simulink model "SMIB_with_DFIG_IO"  (R2016a)
settings: Solver=ode4  StartTime=0.0  StopTime=10  FixedStep=0.01  RelTol=1e-3
values from neighbouring files (symbols this model uses):
  d_base = 5.0009990    (= 5.000999)    [find_dfig_state_initial_conditions.m]
  d_Beta = 0    [find_dfig_state_initial_conditions.m]
  d_bl = 40.0595545    [find_dfig_state_initial_conditions.m]
  d_Cdc = 2    [find_dfig_state_initial_conditions.m]
  d_Cf = d_FLTR(6)    [find_dfig_state_initial_conditions.m]
  d_ctg = 0.01    [Initialising_SMIB_DFIG.m]    (also in Initialising_two_area_DFIG.m; find_dfig_state_initial_conditions.m = data_DF(10))
  d_esd = -d_Kmrr.*d_ws.*(d_Lrr.*d_irq + d_Lm.*d_isq)    [find_dfig_state_initial_conditions.m]
  d_esq = d_Kmrr.*d_ws.*(d_Lrr.*d_ird + d_Lm.*d_isd)    [find_dfig_state_initial_conditions.m]
  d_GSC_IL1_iv = real(d_vi_dash)    [find_dfig_state_initial_conditions.m]
  d_GSC_IL1_kp = 0.3    [Initialising_SMIB_DFIG.m]    (also in Initialising_two_area_DFIG.m)
  d_GSC_IL2_iv = imag(d_vi_dash)    [find_dfig_state_initial_conditions.m]
  d_GSC_IL2_kp = 0.3    [Initialising_SMIB_DFIG.m]    (also in Initialising_two_area_DFIG.m)
  d_GSC_OL1_iv = real(d_ii_dash)    [find_dfig_state_initial_conditions.m]
  d_GSC_OL1_kp = -22    [Initialising_SMIB_DFIG.m]    (also in Initialising_two_area_DFIG.m)
  d_GSC_OL2_iv = imag(d_ii_dash)    [find_dfig_state_initial_conditions.m]
  d_GSC_OL2_kp = 0    [Initialising_SMIB_DFIG.m]    (also in Initialising_two_area_DFIG.m)
  d_Hg = 0.4    [Initialising_SMIB_DFIG.m]    (also in Initialising_two_area_DFIG.m; find_dfig_state_initial_conditions.m = data_DF(12))
  d_Ht = 4    [Initialising_SMIB_DFIG.m]    (also in Initialising_two_area_DFIG.m; find_dfig_state_initial_conditions.m = data_DF(11))
  d_igd = xdfig(:,10)    [find_dfig_state_initial_conditions.m]
  d_igq = xdfig(:,9)    [find_dfig_state_initial_conditions.m]
  d_iid = xdfig(:,8)    [find_dfig_state_initial_conditions.m]
  d_iiq = xdfig(:,7)    [find_dfig_state_initial_conditions.m]
  d_isd = xdfig(:,2)    [find_dfig_state_initial_conditions.m]
  d_isq = xdfig(:,1)    [find_dfig_state_initial_conditions.m]
  d_Kmrr = d_Lm/d_Lrr    [find_dfig_state_initial_conditions.m]
  d_Kopt = 1    [Initialising_SMIB_DFIG.m]    (also in Initialising_two_area_DFIG.m; find_dfig_state_initial_conditions.m = data_DF(8))
  d_ktg = 0.3    [Initialising_SMIB_DFIG.m]    (also in Initialising_two_area_DFIG.m)
  d_Lg = d_FLTR(5)    [find_dfig_state_initial_conditions.m]
  d_Li = d_FLTR(4)    [find_dfig_state_initial_conditions.m]
  d_Lm = 4    [Initialising_SMIB_DFIG.m]    (also in Initialising_two_area_DFIG.m; find_dfig_state_initial_conditions.m = data_DF(3))
  d_Ls_d = d_Lss - (d_Lm^2/d_Lrr)    [find_dfig_state_initial_conditions.m]
  d_MSC_IL1_iv = 0.0389    [Initialising_SMIB_DFIG.m]    (also in Initialising_two_area_DFIG.m; find_dfig_state_initial_conditions.m = real(d_vr_dash))
  d_MSC_IL1_kp = -0.23    [Initialising_SMIB_DFIG.m]    (also in Initialising_two_area_DFIG.m)
  d_MSC_IL2_iv = imag(d_vr_dash)    [find_dfig_state_initial_conditions.m]
  d_MSC_IL2_kp = -0.23    [Initialising_SMIB_DFIG.m]    (also in Initialising_two_area_DFIG.m)
  d_MSC_OL1_iv = real(d_ir_dash)    [find_dfig_state_initial_conditions.m]
  d_MSC_OL1_kp = 0    [Initialising_SMIB_DFIG.m]    (also in Initialising_two_area_DFIG.m)
  d_MSC_OL2_iv = imag(d_ir_dash)    [find_dfig_state_initial_conditions.m]
  d_MSC_OL2_kp = 0    [Initialising_SMIB_DFIG.m]    (also in Initialising_two_area_DFIG.m)
  d_Qs = Qdfig    [find_dfig_state_initial_conditions.m]
  d_R1 = d_Rs + d_R2    [find_dfig_state_initial_conditions.m]
  d_R2 = d_Kmrr^2*d_Rr    [find_dfig_state_initial_conditions.m]
  d_Rc = d_FLTR(3)    [find_dfig_state_initial_conditions.m]
  d_Rg = 0.0    (= 0)    [find_dfig_state_initial_conditions.m]
  d_Ri = 0.0    (= 0)    [find_dfig_state_initial_conditions.m]
  d_Tr = d_Lrr/d_Rr    [find_dfig_state_initial_conditions.m]
  d_Ts = 0.9386    [find_dfig_state_initial_conditions.m]
  d_vcd = xdfig(:,14)    [find_dfig_state_initial_conditions.m]
  d_vcq = 0.9837    [Initialising_SMIB_DFIG.m]    (also in Initialising_two_area_DFIG.m)
  d_VDC = 1.5    [find_dfig_state_initial_conditions.m]
  d_vw = 14.5316    [Initialising_SMIB_DFIG.m]    (also in Initialising_two_area_DFIG.m; find_dfig_state_initial_conditions.m)
  d_wb = 2*pi*50    (= 314.159265359)    [Initialising_SMIB_DFIG.m]    (also in Initialising_two_area_DFIG.m; find_dfig_state_initial_conditions.m)
  d_welb = 2*pi*50    (= 314.159265359)    [find_dfig_state_initial_conditions.m]
  d_wg = 0.9688    [find_dfig_state_initial_conditions.m]
  d_ws = 1    [Initialising_SMIB_DFIG.m]    (also in Initialising_two_area_DFIG.m; find_dfig_state_initial_conditions.m)
  d_wt = 0.9688    [find_dfig_state_initial_conditions.m]
  d_wtrated = 3.0337    [find_dfig_state_initial_conditions.m]
  d_Xm = d_Lm    [find_dfig_state_initial_conditions.m]
  dfig_mult = zeros(size(bus_sln,1)-1,size(Dmachs,1))    [Initialising_SMIB_DFIG.m]    (also in Initialising_two_area_DFIG.m)
  ExpandSmachs = [1]    [Initialising_SMIB_DFIG.m]    (also in Initialising_two_area_DFIG.m)
  MMST_mult = zeros(size(bus_sln,1)-1,size(Smachs,1))    [Initialising_SMIB_DFIG.m]    (also in Initialising_two_area_DFIG.m)
  rho = 1.225    [find_dfig_state_initial_conditions.m]
  s_delta = s_delta*(180/pi)    [Initialising_SMIB_DFIG.m]    (also in Initialising_two_area_DFIG.m; generic_Sync_Init.m = angle(s_Eq))
  s_Edd = -(s_xq-s_xqd).* s_iq    [generic_Sync_Init.m]
  s_Efd = abs(s_Eq) - (s_xd-s_xq).*s_id    [generic_Sync_Init.m]
  s_Eqd = s_Efd + (s_xd-s_xdd).*s_id    [generic_Sync_Init.m]
  s_f = 60    [generic_Sync_Init.m]
  s_Ka = 200    [two_area_synch.m]
  s_Psi2q = -s_Edd+(s_xqd-s_xls).*s_iq    [generic_Sync_Init.m]
  s_Psild = s_Eqd+(s_xdd-s_xls).*s_id    [generic_Sync_Init.m]
  s_Rgov = 0.05    [two_area_synch.m]
  s_Ta = 0.02    [two_area_synch.m]
  s_Tg = 0.2    [two_area_synch.m]
  s_Tm = s_Te    [generic_Sync_Init.m]
  s_Vref = s_volt+1./s_Ka.*s_Efd    [generic_Sync_Init.m]
  s_ws = 0    [generic_Sync_Init.m]
  SelectSmachs = [1]    [Initialising_SMIB_DFIG.m]    (also in Initialising_two_area_DFIG.m)
  small_d = [ ... (first row only)    [Initialising_SMIB_DFIG.m]    (also in Initialising_two_area_DFIG.m; initSSA.m; two_area_synch.m)
  vinf = bus_sln(3,2)*exp(1i*bus_sln(3,3)*pi/180)    [Initialising_SMIB_DFIG.m]    (also in Initialising_two_area_DFIG.m)
  ZA = Znet(1:end-1,1:end-1)    [Initialising_SMIB_DFIG.m]    (also in Initialising_two_area_DFIG.m)
  ZB = Znet(1:end-1,end)    [Initialising_SMIB_DFIG.m]    (also in Initialising_two_area_DFIG.m)
  ZC = Znet(end,1:end-1)    [Initialising_SMIB_DFIG.m]    (also in Initialising_two_area_DFIG.m)
  ZD = Znet(end,end)    [Initialising_SMIB_DFIG.m]    (also in Initialising_two_area_DFIG.m)
undefined symbols (not defined in the file or in its folder): j, s_D, s_H, s_Rs, s_Tdod, s_Tdodd, s_Tqod, s_Tqodd, s_xd, s_xdd, s_xddd, s_xls, s_xq, s_xqd, s_xqdd
libraries: powerlib_extras x1
settings Model: Creator=EBUKA  LastModifiedBy=EBUKA
settings GRTTargetCC: GeneratePreprocessorConditionals=Use local settings

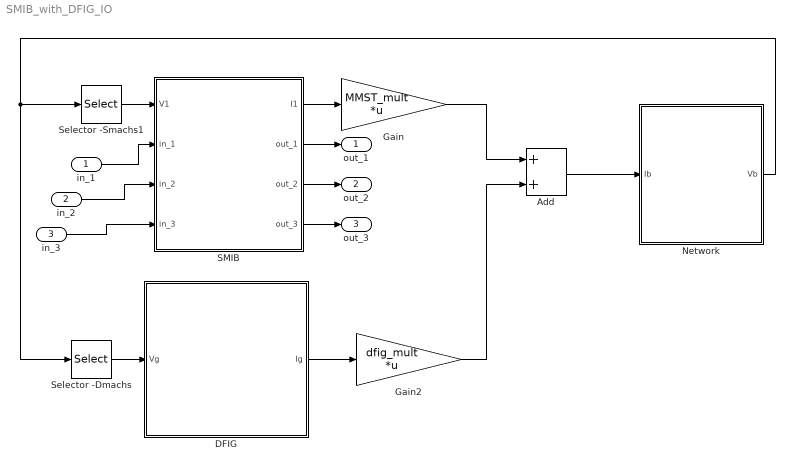
== system SMIB_with_DFIG_IO ==
  in_1 : Inport
  in_2 : Inport  Port=2
  in_3 : Inport  Port=3
  Add : Sum
  DFIG : Subsystem
  Gain : Gain  Gain=MMST_mult  Multiplication=Matrix(K*u)
  Gain2 : Gain  Gain=dfig_mult  Multiplication=Matrix(K*u)
  Network : Subsystem
  SMIB : Subsystem
  Selector -Dmachs : Selector  InputPortWidth=13  IndexOptions=Index vector (dialog)  Indices=Dmachs  OutputSizes=1
  Selector -Smachs1 : Selector  InputPortWidth=13  IndexOptions=Index vector (dialog)  Indices=Smachs  OutputSizes=1
  out_1 : Outport
  out_2 : Outport  Port=2
  out_3 : Outport  Port=3
  wires:
  Selector -Smachs1/1 -> SMIB/1(V1)
  SMIB/1(I1) -> Gain/1
  Add/1 -> Network/1(Ib)
  Gain/1 -> Add/1
  Gain2/1 -> Add/2
  DFIG/1(Ig) -> Gain2/1
  Selector -Dmachs/1 -> DFIG/1(Vg)
  Network/1(Vb) -> Selector -Smachs1/1, Selector -Dmachs/1
  in_1/1 -> SMIB/2(in_1)
  in_2/1 -> SMIB/3(in_2)
  in_3/1 -> SMIB/4(in_3)
  SMIB/2(out_1) -> out_1/1
  SMIB/3(out_2) -> out_2/1
  SMIB/4(out_3) -> out_3/1

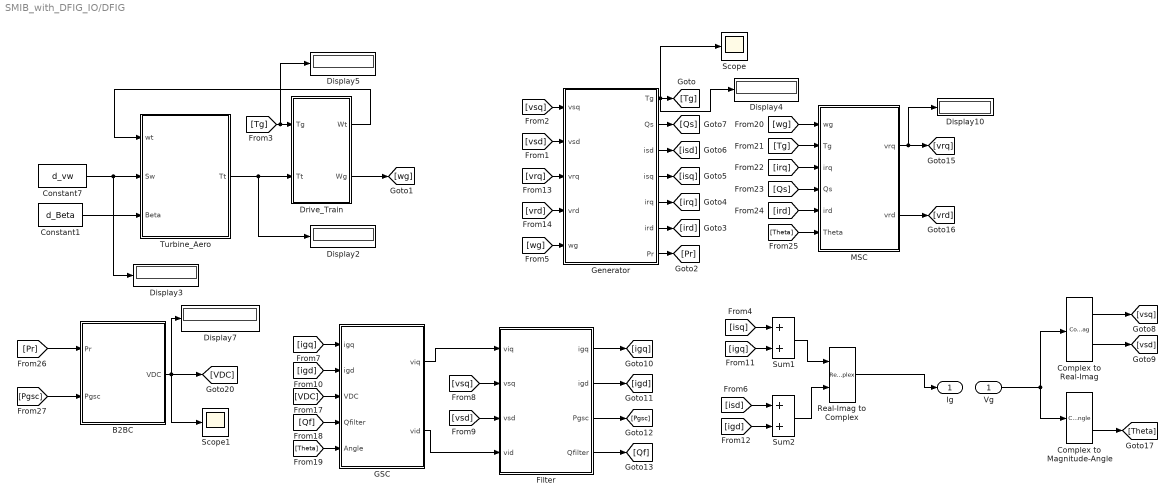
== system SMIB_with_DFIG_IO/DFIG ==
  Vg : Inport
  B2BC : Subsystem
  Complex to Magnitude-Angle : ComplexToMagnitudeAngle
  Complex to Real-Imag : ComplexToRealImag
  Constant1 : Constant  Value=d_Beta
  Constant7 : Constant  Value=d_vw
  Display{2..5,7,10} (6 alike) : Display
  Drive_Train : Subsystem
  Filter : Subsystem
  GSC : Subsystem
  Generator : Subsystem
  MSC : Subsystem
  Real-Imag to Complex : RealImagToComplex
  Scope : Scope
  Scope1 : Scope
  Sum1 : Sum
  Sum2 : Sum
  Turbine_Aero : Subsystem
  Ig : Outport
  wires:
  [vrd] -> Generator/4(vrd)
  [vsd] -> Generator/2(vsd)
  Drive_Train/1(Wt) -> Turbine_Aero/1(wt)
  Generator/6(ird) -> [ird]
  [Tg] -> Display5/1, Drive_Train/1(Tg)
  Constant7/1 -> Display3/1, Turbine_Aero/2(Sw)
  Turbine_Aero/1(Tt) -> Display2/1, Drive_Train/2(Tt)
  [wg] -> Generator/5(wg)
  Generator/1(Tg) -> Display4/1, Scope/1, [Tg]
  Drive_Train/2(Wg) -> [wg]
  [vrq] -> Generator/3(vrq)
  Constant1/1 -> Turbine_Aero/3(Beta)
  Generator/5(irq) -> [irq]
  [Qs] -> MSC/4(Qs)
  [igq] -> GSC/1(igq)
  [Qf] -> GSC/4(Qfilter)
  [vsq] -> Generator/1(vsq)
  [Tg] -> MSC/2(Tg)
  Generator/4(isq) -> [isq]
  [ird] -> MSC/5(ird)
  [vsq] -> Filter/2(vsq)
  Generator/3(isd) -> [isd]
  Generator/2(Qs) -> [Qs]
  Filter/1(igq) -> [igq]
  Filter/2(igd) -> [igd]
  Filter/4(Qfilter) -> [Qf]
  [igd] -> GSC/2(igd)
  [VDC] -> GSC/3(VDC)
  [Theta] -> GSC/5(Angle)
  [wg] -> MSC/1(wg)
  [irq] -> MSC/3(irq)
  [Theta] -> MSC/6(Theta)
  [vsd] -> Filter/3(vsd)
  [Pgsc] -> B2BC/2(Pgsc)
  B2BC/1(VDC) -> Scope1/1, [VDC], Display7/1
  GSC/1(viq) -> Filter/1(viq)
  Filter/3(Pgsc) -> [Pgsc]
  MSC/2(vrd) -> [vrd]
  GSC/2(vid) -> Filter/4(vid)
  MSC/1(vrq) -> Display10/1, [vrq]
  [Pr] -> B2BC/1(Pr)
  Generator/7(Pr) -> [Pr]
  Complex to Magnitude-Angle/2 -> [Theta]
  [isq] -> Sum1/1
  Sum2/1 -> Real-Imag to Complex/2
  [isd] -> Sum2/1
  [igd] -> Sum2/2
  Complex to Real-Imag/2 -> [vsd]
  Complex to Real-Imag/1 -> [vsq]
  [igq] -> Sum1/2
  Sum1/1 -> Real-Imag to Complex/1
  Vg/1 -> Complex to Magnitude-Angle/1, Complex to Real-Imag/1
  Real-Imag to Complex/1 -> Ig/1

== system SMIB_with_DFIG_IO/Network ==
  Ib : Inport
  Constant5 : Constant  Value=vinf
  Gain1 : Gain  Gain=ZA-ZB*inv(ZD)*ZC  Multiplication=Matrix(K*u)
  Gain2 : Gain  Gain=ZB*inv(ZD)  Multiplication=Matrix(K*u)
  Sum3 : Sum
  Vb : Outport
  wires:
  Ib/1 -> Gain1/1
  Gain1/1 -> Sum3/1
  Sum3/1 -> Vb/1
  Gain2/1 -> Sum3/2
  Constant5/1 -> Gain2/1

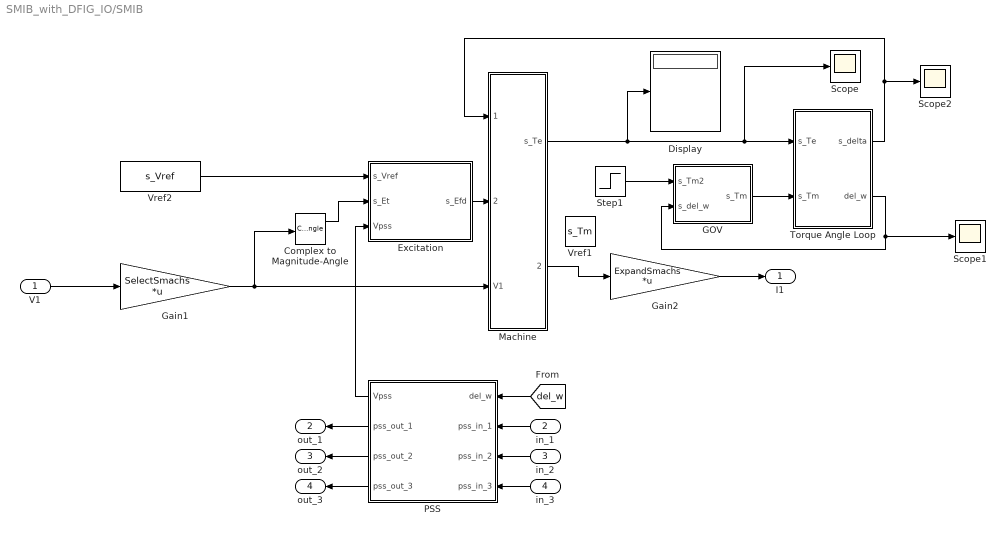
== system SMIB_with_DFIG_IO/SMIB ==
  V1 : Inport
  in_1 : Inport  Port=2
  in_2 : Inport  Port=3
  in_3 : Inport  Port=4
  Complex to Magnitude-Angle : ComplexToMagnitudeAngle
  Display : Display
  Excitation : Subsystem
  GOV : Subsystem
  Gain1 : Gain  Gain=SelectSmachs  Multiplication=Matrix(K*u)
  Gain2 : Gain  Gain=ExpandSmachs  Multiplication=Matrix(K*u)
  Machine : Subsystem
  PSS : Subsystem
  Scope : Scope
  Scope1 : Scope
  Scope2 : Scope
  Step1 : Step  Before=s_Tm  After=s_Tm+0.07031  SampleTime=0
  Torque Angle Loop : Subsystem
  Vref1 : Constant  Value=s_Tm
  Vref2 : Constant  Value=s_Vref
  I1 : Outport
  out_1 : Outport  Port=2
  out_2 : Outport  Port=3
  out_3 : Outport  Port=4
  wires:
  Gain1/1 -> Machine/3(V1), Complex to Magnitude-Angle/1
  Gain2/1 -> I1/1
  Torque Angle Loop/1(s_delta) -> Scope2/1, Machine/1(s_delta)
  Machine/2(s_iDQ) -> Gain2/1
  Torque Angle Loop/2(del_w) -> Scope1/1, GOV/2(s_del_w)
  Complex to Magnitude-Angle/1 -> Excitation/2(s_Et)
  Machine/1(s_Te) -> Display/1, Scope/1, Torque Angle Loop/1("s_Te ")
  GOV/1(s_Tm) -> Torque Angle Loop/2(s_Tm)
  Step1/1 -> GOV/1(s_Tm2)
  Excitation/1(s_Efd) -> Machine/2(s_Efd)
  Vref2/1 -> Excitation/1(s_Vref)
  V1/1 -> Gain1/1
  PSS/1(Vpss) -> Excitation/3(Vpss)
  PSS/2(pss_out_1) -> out_1/1
  PSS/3(pss_out_2) -> out_2/1
  PSS/4(pss_out_3) -> out_3/1
  [del_w] -> PSS/1(del_w)
  in_1/1 -> PSS/2(pss_in_1)
  in_2/1 -> PSS/3(pss_in_2)
  in_3/1 -> PSS/4(pss_in_3)

== system SMIB_with_DFIG_IO/DFIG/B2BC ==
  Pr : Inport
  Pgsc : Inport  Port=2
  Add : Sum  Inputs=+-
  Gain : Gain  Gain=1/d_Cdc
  Gain4 : Gain  Gain=1/d_VDC
  Gain5 : Gain  Gain=1/d_VDC
  VDC : Outport
  wires:
  Add/1 -> Gain/1
  Gain4/1 -> Add/1
  Pr/1 -> Gain4/1
  Gain5/1 -> Add/2
  Pgsc/1 -> Gain5/1
  Gain/1 -> VDC/1

== system SMIB_with_DFIG_IO/DFIG/Drive_Train ==
  Tg : Inport
  Tt : Inport  Port=2
  Add : Sum  Inputs=-+
  Add1 : Sum  Inputs=+-
  Add2 : Sum  Inputs=-+
  Add3 : Sum
  Gain : Gain  Gain=1./(2*d_Hg)
  Gain1 : Gain  Gain=1./(2*d_Ht)
  Gain2 : Gain  Gain=d_welb
  Gain3 : Gain  Gain=d_ktg
  Gain4 : Gain  Gain=d_ctg
  d_Ts : Integrator  InitialCondition=d_Ts
  d_wg : Integrator  InitialCondition=d_wg
  d_wt : Integrator  InitialCondition=d_wt
  Wt : Outport
  Wg : Outport  Port=2
  wires:
  Gain1/1 -> d_wt/1
  Add3/1 -> Add1/2, Add/2
  Tt/1 -> Add1/1
  Add/1 -> Gain/1
  d_wt/1 -> Wt/1, Add2/2
  d_Ts/1 -> Add3/1
  d_wg/1 -> Wg/1, Add2/1
  Gain3/1 -> d_Ts/1
  Tg/1 -> Add/1
  Gain2/1 -> Gain4/1, Gain3/1
  Add1/1 -> Gain1/1
  Gain4/1 -> Add3/2
  Add2/1 -> Gain2/1
  Gain/1 -> d_wg/1

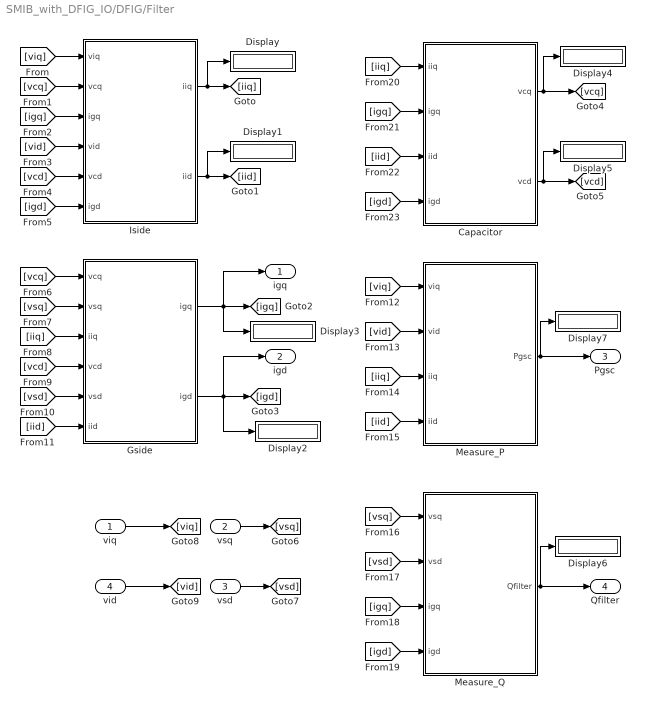
== system SMIB_with_DFIG_IO/DFIG/Filter ==
  viq : Inport
  vsq : Inport  Port=2
  vsd : Inport  Port=3
  vid : Inport  Port=4
  Capacitor : Subsystem
  Display{,1..7} (8 alike) : Display
  Gside : Subsystem
  Iside : Subsystem
  Measure_P : Subsystem
  Measure_Q : Subsystem
  igq : Outport
  igd : Outport  Port=2
  Pgsc : Outport  Port=3
  Qfilter : Outport  Port=4
  wires:
  [viq] -> Iside/1(viq)
  [vid] -> Iside/4(vid)
  [igd] -> Iside/6(igd)
  [iiq] -> Gside/3(iiq)
  Gside/2(igd) -> igd/1, Display2/1, [igd]
  [iiq] -> Capacitor/1(iiq)
  Capacitor/2(vcd) -> [vcd], Display5/1
  [iid] -> Capacitor/3(iid)
  [vcd] -> Gside/4(vcd)
  [vsd] -> Gside/5(vsd)
  [igd] -> Capacitor/4(igd)
  [vcq] -> Gside/1(vcq)
  [iid] -> Gside/6(iid)
  [vcd] -> Iside/5(vcd)
  [vsq] -> Gside/2(vsq)
  [vcq] -> Iside/2(vcq)
  [igq] -> Iside/3(igq)
  [igq] -> Capacitor/2(igq)
  Capacitor/1("vcq ") -> [vcq], Display4/1
  vid/1 -> [vid]
  vsq/1 -> [vsq]
  Iside/1(iiq) -> Display/1, [iiq]
  [vsd] -> Measure_Q/2(vsd)
  [viq] -> Measure_P/1(viq)
  [vid] -> Measure_P/2(vid)
  [iiq] -> Measure_P/3(iiq)
  viq/1 -> [viq]
  Iside/2(iid) -> Display1/1, [iid]
  [igq] -> Measure_Q/3("igq ")
  [vsq] -> Measure_Q/1(vsq)
  Gside/1(igq) -> igq/1, Display3/1, [igq]
  [iid] -> Measure_P/4(iid)
  Measure_Q/1(Qfilter) -> Qfilter/1, Display6/1
  [igd] -> Measure_Q/4(igd)
  vsd/1 -> [vsd]
  Measure_P/1(Pgsc) -> Pgsc/1, Display7/1

== system SMIB_with_DFIG_IO/DFIG/GSC ==
  igq : Inport
  igd : Inport  Port=2
  VDC : Inport  Port=3
  Qfilter : Inport  Port=4
  Angle : Inport  Port=5
  Add10 : Sum  Inputs=-+
  Add7 : Sum  Inputs=+-
  Add8 : Sum  Inputs=+-
  Add9 : Sum  Inputs=-+
  Constant8 : Constant  Value=0
  Constant9 : Constant  Value=d_VDC
  GSC_IL1 : Subsystem
  GSC_IL2 : Subsystem
  GSC_OL1 : Subsystem
  GSC_OL2 : Subsystem
  MSC_OL7 : Subsystem
  MSC_OL8 : Subsystem
  viq : Outport
  vid : Outport  Port=2
  wires:
  Add7/1 -> GSC_OL1/1(In1)
  Constant9/1 -> Add7/1
  Add9/1 -> GSC_IL2/1(In1)
  Add10/1 -> GSC_OL2/1(In1)
  Add8/1 -> GSC_IL1/1(In1)
  GSC_OL2/1(iDref) -> Add9/2
  Constant8/1 -> Add10/2
  VDC/1 -> Add7/2
  GSC_OL1/1(iQref) -> Add8/1
  Angle/1 -> MSC_OL8/3(Angle), MSC_OL7/3(Angle)
  Qfilter/1 -> Add10/1
  igq/1 -> MSC_OL7/1(iQ)
  igd/1 -> MSC_OL7/2(iD)
  MSC_OL7/1(iQ') -> Add8/2
  MSC_OL7/2(iD') -> Add9/1
  GSC_IL1/1(vQref) -> MSC_OL8/1(VQ')
  GSC_IL2/1(vDref) -> MSC_OL8/2(VD')
  MSC_OL8/1(VQ) -> viq/1
  MSC_OL8/2(VD) -> vid/1

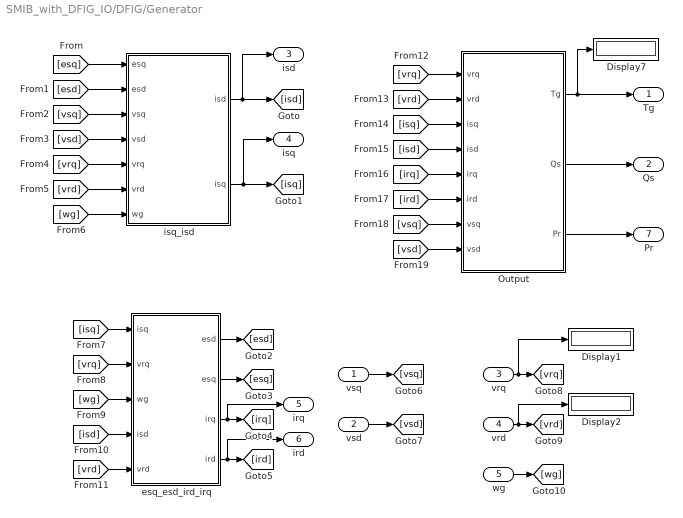
== system SMIB_with_DFIG_IO/DFIG/Generator ==
  vsq : Inport
  vsd : Inport  Port=2
  vrq : Inport  Port=3
  vrd : Inport  Port=4
  wg : Inport  Port=5
  Display1 : Display
  Display2 : Display
  Display7 : Display
  Output : Subsystem
  esq_esd_ird_irq : Subsystem
  isq_isd : Subsystem
  Tg : Outport
  Qs : Outport  Port=2
  isd : Outport  Port=3
  isq : Outport  Port=4
  irq : Outport  Port=5
  ird : Outport  Port=6
  Pr : Outport  Port=7
  wires:
  [vrd] -> esq_esd_ird_irq/5(vrd)
  esq_esd_ird_irq/3(irq) -> [irq], irq/1
  Output/3(Pr) -> Pr/1
  esq_esd_ird_irq/4(ird) -> ird/1, [ird]
  [wg] -> esq_esd_ird_irq/3(wg)
  [vrq] -> esq_esd_ird_irq/2(vrq)
  isq_isd/1(isd) -> isd/1, [isd]
  [wg] -> isq_isd/7(wg)
  [vsq] -> isq_isd/3(vsq)
  [isq] -> esq_esd_ird_irq/1(isq)
  [isd] -> esq_esd_ird_irq/4(isd)
  [vsd] -> isq_isd/4(vsd)
  [isq] -> Output/3(isq)
  [vrd] -> Output/2(vrd)
  [vsq] -> Output/7(vsq)
  [irq] -> Output/5(irq)
  [isd] -> Output/4(isd)
  Output/2(Qs) -> Qs/1
  [vrq] -> Output/1(vrq)
  isq_isd/2(isq) -> isq/1, [isq]
  esq_esd_ird_irq/2(esq) -> [esq]
  [vrq] -> isq_isd/5(vrq)
  esq_esd_ird_irq/1(esd) -> [esd]
  [esd] -> isq_isd/2(esd)
  [esq] -> isq_isd/1(esq)
  [vrd] -> isq_isd/6(vrd)
  Output/1(Tg) -> Tg/1, Display7/1
  [vsd] -> Output/8(vsd)
  [ird] -> Output/6(ird)
  vsq/1 -> [vsq]
  vsd/1 -> [vsd]
  vrq/1 -> Display1/1, [vrq]
  vrd/1 -> Display2/1, [vrd]
  wg/1 -> [wg]

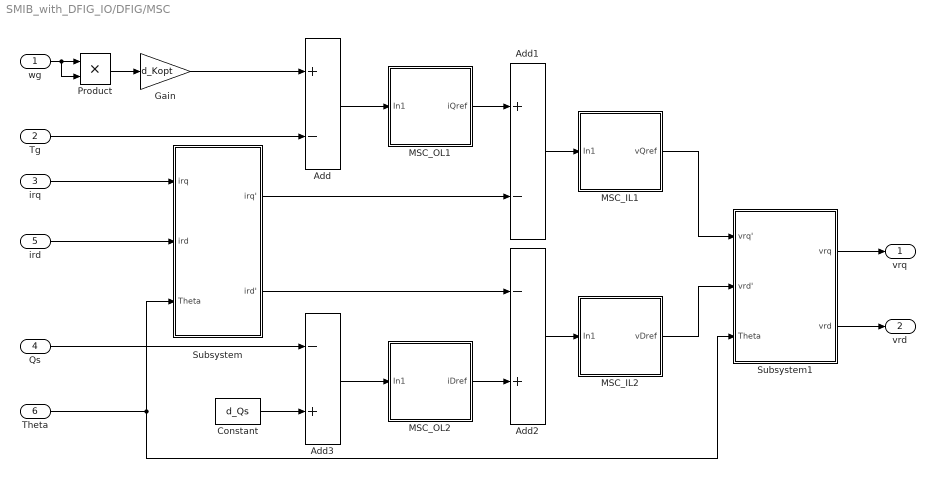
== system SMIB_with_DFIG_IO/DFIG/MSC ==
  wg : Inport
  Tg : Inport  Port=2
  irq : Inport  Port=3
  Qs : Inport  Port=4
  ird : Inport  Port=5
  Theta : Inport  Port=6
  Add : Sum  Inputs=+-
  Add1 : Sum  Inputs=+-
  Add2 : Sum  Inputs=-+
  Add3 : Sum  Inputs=-+
  Constant : Constant  Value=d_Qs
  Gain : Gain  Gain=d_Kopt
  MSC_IL1 : Subsystem
  MSC_IL2 : Subsystem
  MSC_OL1 : Subsystem
  MSC_OL2 : Subsystem
  Product : Product
  Subsystem : Subsystem
  Subsystem1 : Subsystem
  vrq : Outport
  vrd : Outport  Port=2
  wires:
  Product/1 -> Gain/1
  wg/1 -> Product/2, Product/1
  Gain/1 -> Add/1
  Tg/1 -> Add/2
  irq/1 -> Subsystem/1(irq)
  Add/1 -> MSC_OL1/1(In1)
  MSC_OL1/1(iQref) -> Add1/1
  Subsystem/1(irq') -> Add1/2
  MSC_OL2/1(iDref) -> Add2/2
  Subsystem/2(ird') -> Add2/1
  Add3/1 -> MSC_OL2/1(In1)
  Constant/1 -> Add3/2
  Qs/1 -> Add3/1
  ird/1 -> Subsystem/2(ird)
  Add1/1 -> MSC_IL1/1(In1)
  Add2/1 -> MSC_IL2/1(In1)
  MSC_IL2/1(vDref) -> Subsystem1/2(vrd')
  MSC_IL1/1(vQref) -> Subsystem1/1(vrq')
  Theta/1 -> Subsystem1/3(Theta), Subsystem/3(Theta)
  Subsystem1/1(vrq) -> vrq/1
  Subsystem1/2(vrd) -> vrd/1

== system SMIB_with_DFIG_IO/DFIG/Turbine_Aero ==
  wt : Inport
  Sw : Inport  Port=2
  Beta : Inport  Port=3
  Constant2 : Constant  Value=3
  Constant4 : Constant  Value=0.5*rho*pi*d_bl^2
  Cp_Calc : Subsystem
  Divide1 : Product  Inputs=/*
  Divide2 : Product  Inputs=*/
  Gain1 : Gain  Gain=d_wtrated*d_bl
  Gain2 : Gain  Gain=1/(d_base*10^6)
  Math Function : Math  Operator=pow  SaturateOnIntegerOverflow=on
  Product : Product  Inputs=3
  Tt : Outport
  wires:
  Gain2/1 -> Divide1/2
  Product/1 -> Gain2/1
  Divide1/1 -> Tt/1
  Beta/1 -> Cp_Calc/2(Beta)
  Sw/1 -> Math Function/1, Divide2/2
  Cp_Calc/1(Cp) -> Product/2
  Divide2/1 -> Cp_Calc/1(Lambda)
  Constant2/1 -> Math Function/2
  Constant4/1 -> Product/1
  wt/1 -> Divide1/1, Gain1/1
  Gain1/1 -> Divide2/1
  Math Function/1 -> Product/3

== system SMIB_with_DFIG_IO/SMIB/Excitation ==
  s_Vref : Inport
  s_Et : Inport  Port=2
  Vpss : Inport  Port=3
  1/Tpd2 : Gain  Gain=s_Ka
  1/Tpq1 : Gain  Gain=1./s_Ta
  Constant1 : Constant  Value=s_Efd./s_Ka  VectorParams1D=off
  Integrator2 : Integrator  InitialConditionSource=external
  Product3 : Product  RndMeth=Zero
  Subtract2 : Sum  Inputs=+-
  Subtract5 : Sum  Inputs=+-+
  small_d : powerlib_extras/Control  Blocks/Timer  t=small_d(1,:)  e=small_d(2,:)
  s_Efd : Outport
  wires:
  Constant1/1 -> Integrator2/2
  Subtract2/1 -> 1/Tpq1/1
  1/Tpq1/1 -> Integrator2/1
  Integrator2/1 -> s_Efd/1, Subtract2/2
  Subtract5/1 -> 1/Tpd2/1
  1/Tpd2/1 -> Subtract2/1
  small_d/1 -> Product3/2
  Product3/1 -> Subtract5/1
  s_Vref/1 -> Product3/1
  Vpss/1 -> Subtract5/3
  s_Et/1 -> Subtract5/2

== system SMIB_with_DFIG_IO/SMIB/GOV ==
  s_Tm2 : Inport
  s_del_w : Inport  Port=2
  Display : Display
  Gain : Gain  Gain=1./s_Tg
  Gain4 : Gain  Gain=1./s_Rgov
  Scope : Scope
  Scope2 : Scope
  Sum : Sum  Inputs=|+-
  Sum1 : Sum  Inputs=|+-
  s_Tm1 : Integrator  InitialCondition=s_Tm
  s_Tm : Outport
  wires:
  s_Tm2/1 -> Scope/1, Display/1, Sum/1
  s_del_w/1 -> Gain4/1
  Gain4/1 -> Sum/2
  Sum/1 -> Sum1/1
  Sum1/1 -> Gain/1
  Gain/1 -> s_Tm1/1
  s_Tm1/1 -> Sum1/2, Scope2/1, s_Tm/1

== system SMIB_with_DFIG_IO/SMIB/Machine ==
  s_delta : Inport
  s_Efd : Inport  Port=2
  V1 : Inport  Port=3
  DQ to dq : Subsystem
  Machine Equations : Subsystem
  Mathematical block : Subsystem
  dq to DQ : Subsystem
  s_Te : Outport
  s_iDQ : Outport  Port=2
  wires:
  s_Efd/1 -> Machine Equations/1(s_Efd)
  Machine Equations/1(s_Te) -> s_Te/1
  Machine Equations/2(s_iq) -> dq to DQ/1(s_iq)
  Machine Equations/3(s_id) -> dq to DQ/2(s_id)
  V1/1 -> DQ to dq/1(V1)
  DQ to dq/1("s_vq ") -> Machine Equations/3(s_vq)
  DQ to dq/2(s_vd) -> Machine Equations/2(s_vd)
  s_delta/1 -> Mathematical block/1(s_delta)
  Mathematical block/1(exp(-j*s_delta)) -> DQ to dq/2(exp(-j*s_delta))
  Mathematical block/2(exp(j*s_delta)) -> dq to DQ/3(exp(j*s_delta))
  dq to DQ/1(s_iDQ) -> s_iDQ/1

== system SMIB_with_DFIG_IO/SMIB/PSS ==
  del_w : Inport
  pss_in_1 : Inport  Port=2
  pss_in_2 : Inport  Port=3
  pss_in_3 : Inport  Port=4
  1/Tpd1 : Gain  Gain=1/s_ws
  1/Tpd2 : Gain  Gain=1/s_ws
  1/Tpd3 : Gain  Gain=1/s_ws
  Constant1 : Constant  Value=s_ws  VectorParams1D=off
  Constant2 : Constant  Value=0  VectorParams1D=off
  Id1 : Selector  InputPortWidth=4  IndexOptions=Index vector (dialog)  Indices=[2]  OutputSizes=1
  Id2 : Selector  InputPortWidth=4  IndexOptions=Index vector (dialog)  Indices=[4]  OutputSizes=1
  Id3 : Selector  InputPortWidth=4  IndexOptions=Index vector (dialog)  Indices=[1]  OutputSizes=1
  Mux2 : Mux
  Subtract1 : Sum  Inputs=+-
  Subtract2 : Sum  Inputs=+-
  Subtract5 : Sum  Inputs=+-
  Vpss : Outport
  pss_out_1 : Outport  Port=2
  pss_out_2 : Outport  Port=3
  pss_out_3 : Outport  Port=4
  wires:
  Subtract5/1 -> 1/Tpd2/1
  Mux2/1 -> Vpss/1
  1/Tpd2/1 -> pss_out_1/1
  Id3/1 -> Subtract5/1
  Subtract1/1 -> 1/Tpd1/1
  1/Tpd1/1 -> pss_out_2/1
  Id1/1 -> Subtract1/1
  del_w/1 -> Id3/1, Id2/1, Id1/1
  Constant1/1 -> Subtract5/2, Subtract2/2, Subtract1/2
  Subtract2/1 -> 1/Tpd3/1
  1/Tpd3/1 -> pss_out_3/1
  Id2/1 -> Subtract2/1
  pss_in_1/1 -> Mux2/1
  pss_in_2/1 -> Mux2/2
  Constant2/1 -> Mux2/3
  pss_in_3/1 -> Mux2/4

== system SMIB_with_DFIG_IO/SMIB/Torque Angle Loop ==
  "s_Te " : Inport
  s_Tm : Inport  Port=2
  Add : Sum  Inputs=+--
  Add1 : Sum  Inputs=-+
  Constant1 : Constant  Value=s_ws
  Gain : Gain  Gain=2*pi*s_H
  Gain1 : Gain  Gain=180/pi
  Gain2 : Gain  Gain=s_D
  Gain4 : Gain  Gain=1/(2*pi*s_f)
  Integrator2 : Integrator  InitialCondition=s_ws
  Integrator3 : Integrator  InitialCondition=s_delta
  Scope1 : Scope
  Scope2 : Scope
  s_delta : Outport
  del_w : Outport  Port=2
  tag scope: del_w=global
  wires:
  "s_Te "/1 -> Add/2
  Add/1 -> Gain/1
  Gain/1 -> Integrator2/1
  Gain2/1 -> Add/3
  Integrator2/1 -> Add1/2
  Constant1/1 -> Add1/1
  Add1/1 -> Gain2/1, Gain4/1, Scope2/1, Integrator3/1
  s_Tm/1 -> Add/1
  Integrator3/1 -> Gain1/1, s_delta/1
  Gain4/1 -> Scope1/1, [del_w], del_w/1
  Gain1/1 -> [s_delta]

== system SMIB_with_DFIG_IO/DFIG/Filter/Capacitor ==
  iiq : Inport
  igq : Inport  Port=2
  iid : Inport  Port=3
  igd : Inport  Port=4
  Add : Sum  Inputs=+--
  Add1 : Sum  Inputs=+-+
  Gain : Gain  Gain=(d_Cf/d_wb)
  Gain1 : Gain  Gain=(d_wg*d_Cf)
  Gain2 : Gain  Gain=(d_Cf/d_wb)
  Gain3 : Gain  Gain=(d_wg*d_Cf)
  d_vcd : Integrator  InitialCondition=d_vcd
  d_vcq : Integrator  InitialCondition=d_vcq
  "vcq " : Outport
  vcd : Outport  Port=2
  wires:
  d_vcq/1 -> Gain3/1, "vcq "/1
  Add/1 -> Gain/1
  Gain/1 -> d_vcq/1
  iiq/1 -> Add/1
  igq/1 -> Add/2
  Gain1/1 -> Add/3
  d_vcd/1 -> Gain1/1, vcd/1
  Gain2/1 -> d_vcd/1
  Add1/1 -> Gain2/1
  Gain3/1 -> Add1/1
  igd/1 -> Add1/2
  iid/1 -> Add1/3

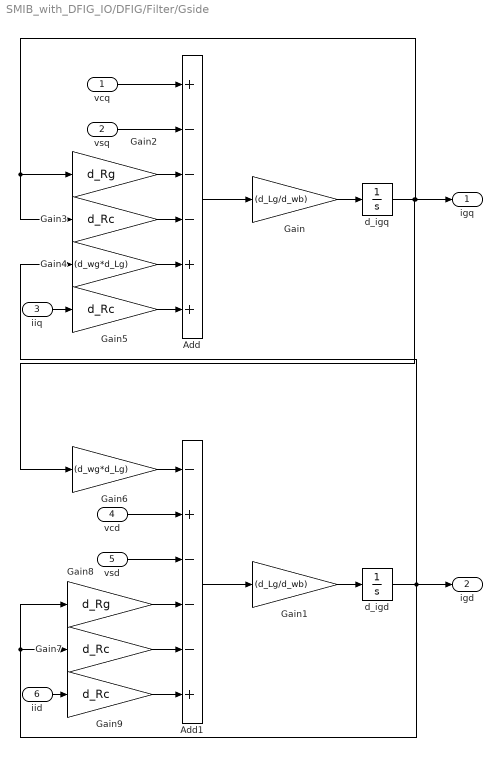
== system SMIB_with_DFIG_IO/DFIG/Filter/Gside ==
  vcq : Inport
  vsq : Inport  Port=2
  iiq : Inport  Port=3
  vcd : Inport  Port=4
  vsd : Inport  Port=5
  iid : Inport  Port=6
  Add : Sum  Inputs=+---++
  Add1 : Sum  Inputs=-+---+
  Gain : Gain  Gain=(d_Lg/d_wb)
  Gain1 : Gain  Gain=(d_Lg/d_wb)
  Gain2 : Gain  Gain=d_Rg
  Gain{3,5,7,9} (4 alike) : Gain  Gain=d_Rc
  Gain4 : Gain  Gain=(d_wg*d_Lg)
  Gain6 : Gain  Gain=(d_wg*d_Lg)
  Gain8 : Gain  Gain=d_Rg
  d_igd : Integrator  InitialCondition=d_igd
  d_igq : Integrator  InitialCondition=d_igq
  igq : Outport
  igd : Outport  Port=2
  wires:
  Gain/1 -> d_igq/1
  Add/1 -> Gain/1
  d_igq/1 -> Gain2/1, Gain3/1, igq/1, Gain6/1
  Gain1/1 -> d_igd/1
  Add1/1 -> Gain1/1
  d_igd/1 -> Gain7/1, Gain8/1, Gain4/1, igd/1
  vcq/1 -> Add/1
  vsq/1 -> Add/2
  Gain2/1 -> Add/3
  Gain3/1 -> Add/4
  Gain4/1 -> Add/5
  Gain5/1 -> Add/6
  iiq/1 -> Gain5/1
  Gain6/1 -> Add1/1
  vcd/1 -> Add1/2
  vsd/1 -> Add1/3
  Gain7/1 -> Add1/5
  Gain8/1 -> Add1/4
  Gain9/1 -> Add1/6
  iid/1 -> Gain9/1

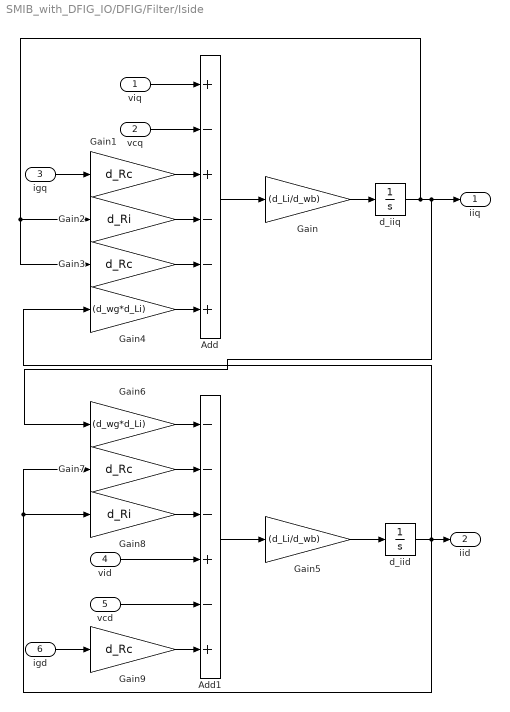
== system SMIB_with_DFIG_IO/DFIG/Filter/Iside ==
  viq : Inport
  vcq : Inport  Port=2
  igq : Inport  Port=3
  vid : Inport  Port=4
  vcd : Inport  Port=5
  igd : Inport  Port=6
  Add : Sum  Inputs=+-+--+
  Add1 : Sum  Inputs=---+-+
  Gain : Gain  Gain=(d_Li/d_wb)
  Gain{1,3,7,9} (4 alike) : Gain  Gain=d_Rc
  Gain2 : Gain  Gain=d_Ri
  Gain4 : Gain  Gain=(d_wg*d_Li)
  Gain5 : Gain  Gain=(d_Li/d_wb)
  Gain6 : Gain  Gain=(d_wg*d_Li)
  Gain8 : Gain  Gain=d_Ri
  d_iid : Integrator  InitialCondition=d_iid
  d_iiq : Integrator  InitialCondition=d_iiq
  iiq : Outport
  iid : Outport  Port=2
  wires:
  Add/1 -> Gain/1
  Gain/1 -> d_iiq/1
  d_iiq/1 -> Gain2/1, Gain3/1, Gain6/1, iiq/1
  viq/1 -> Add/1
  vcq/1 -> Add/2
  Gain1/1 -> Add/3
  igq/1 -> Gain1/1
  Gain2/1 -> Add/4
  Gain3/1 -> Add/5
  Gain4/1 -> Add/6
  Add1/1 -> Gain5/1
  Gain5/1 -> d_iid/1
  d_iid/1 -> Gain7/1, Gain8/1, Gain4/1, iid/1
  Gain6/1 -> Add1/1
  Gain7/1 -> Add1/2
  Gain8/1 -> Add1/3
  vid/1 -> Add1/4
  vcd/1 -> Add1/5
  Gain9/1 -> Add1/6
  igd/1 -> Gain9/1

== system SMIB_with_DFIG_IO/DFIG/Filter/Measure_P ==
  viq : Inport
  vid : Inport  Port=2
  iiq : Inport  Port=3
  iid : Inport  Port=4
  Add : Sum
  Product : Product
  Product1 : Product
  Pgsc : Outport
  wires:
  Add/1 -> Pgsc/1
  Product/1 -> Add/1
  viq/1 -> Product/1
  iiq/1 -> Product/2
  Product1/1 -> Add/2
  vid/1 -> Product1/1
  iid/1 -> Product1/2

== system SMIB_with_DFIG_IO/DFIG/Filter/Measure_Q ==
  vsq : Inport
  vsd : Inport  Port=2
  "igq " : Inport  Port=3
  igd : Inport  Port=4
  Add1 : Sum  Inputs=-+
  Product : Product
  Product1 : Product
  Qfilter : Outport
  wires:
  Add1/1 -> Qfilter/1
  Product/1 -> Add1/1
  Product1/1 -> Add1/2
  vsq/1 -> Product/1
  vsd/1 -> Product1/1
  igd/1 -> Product/2
  "igq "/1 -> Product1/2

== system SMIB_with_DFIG_IO/DFIG/GSC/GSC_IL1 ==
  In1 : Inport
  Gain1 : Gain  Gain=d_GSC_IL1_kp
  Gain2 : Gain  Gain=d_GSC_IL1_kp
  Sum : Sum  Inputs=+|+
  d_GSC_IL1_iv : Integrator  InitialCondition=d_GSC_IL1_iv
  vQref : Outport
  wires:
  Sum/1 -> vQref/1
  In1/1 -> Gain2/1, Gain1/1
  Gain1/1 -> d_GSC_IL1_iv/1
  d_GSC_IL1_iv/1 -> Sum/1
  Gain2/1 -> Sum/2

== system SMIB_with_DFIG_IO/DFIG/GSC/GSC_IL2 ==
  In1 : Inport
  Gain1 : Gain  Gain=d_GSC_IL2_kp
  Gain2 : Gain  Gain=d_GSC_IL2_kp
  Sum : Sum  Inputs=+|+
  d_GSC_IL2_iv : Integrator  InitialCondition=d_GSC_IL2_iv
  vDref : Outport
  wires:
  Sum/1 -> vDref/1
  In1/1 -> Gain2/1, Gain1/1
  Gain1/1 -> d_GSC_IL2_iv/1
  d_GSC_IL2_iv/1 -> Sum/1
  Gain2/1 -> Sum/2

== system SMIB_with_DFIG_IO/DFIG/GSC/GSC_OL1 ==
  In1 : Inport
  Gain1 : Gain  Gain=d_GSC_OL1_kp
  Gain2 : Gain  Gain=d_GSC_OL1_kp
  Sum : Sum  Inputs=+|+
  d_GSC_OL1_iv : Integrator  InitialCondition=d_GSC_OL1_iv
  iQref : Outport
  wires:
  Sum/1 -> iQref/1
  In1/1 -> Gain2/1, Gain1/1
  Gain1/1 -> d_GSC_OL1_iv/1
  d_GSC_OL1_iv/1 -> Sum/1
  Gain2/1 -> Sum/2

== system SMIB_with_DFIG_IO/DFIG/GSC/GSC_OL2 ==
  In1 : Inport
  Gain1 : Gain  Gain=d_GSC_OL2_kp
  Gain2 : Gain  Gain=d_GSC_OL2_kp
  Sum : Sum  Inputs=+|+
  d_GSC_OL2_iv : Integrator  InitialCondition=d_GSC_OL2_iv
  iDref : Outport
  wires:
  Sum/1 -> iDref/1
  In1/1 -> Gain2/1, Gain1/1
  Gain1/1 -> d_GSC_OL2_iv/1
  d_GSC_OL2_iv/1 -> Sum/1
  Gain2/1 -> Sum/2

== system SMIB_with_DFIG_IO/DFIG/GSC/MSC_OL7 ==
  iQ : Inport
  iD : Inport  Port=2
  Angle : Inport  Port=3
  Complex to Real-Imag : ComplexToRealImag
  Gain : Gain  Gain=-j
  Math Function2 : Math  SaturateOnIntegerOverflow=on
  Product : Product
  Real-Imag to Complex : RealImagToComplex
  iQ' : Outport
  iD' : Outport  Port=2
  wires:
  Angle/1 -> Gain/1
  Gain/1 -> Math Function2/1
  Real-Imag to Complex/1 -> Product/1
  Math Function2/1 -> Product/2
  Product/1 -> Complex to Real-Imag/1
  Complex to Real-Imag/1 -> iQ'/1
  Complex to Real-Imag/2 -> iD'/1
  iQ/1 -> Real-Imag to Complex/1
  iD/1 -> Real-Imag to Complex/2

== system SMIB_with_DFIG_IO/DFIG/GSC/MSC_OL8 ==
  VQ' : Inport
  VD' : Inport  Port=2
  Angle : Inport  Port=3
  Complex to Real-Imag : ComplexToRealImag
  Gain1 : Gain  Gain=j
  Math Function2 : Math  SaturateOnIntegerOverflow=on
  Product : Product
  Real-Imag to Complex : RealImagToComplex
  VQ : Outport
  VD : Outport  Port=2
  wires:
  VQ'/1 -> Real-Imag to Complex/1
  VD'/1 -> Real-Imag to Complex/2
  Angle/1 -> Gain1/1
  Gain1/1 -> Math Function2/1
  Real-Imag to Complex/1 -> Product/1
  Math Function2/1 -> Product/2
  Product/1 -> Complex to Real-Imag/1
  Complex to Real-Imag/1 -> VQ/1
  Complex to Real-Imag/2 -> VD/1

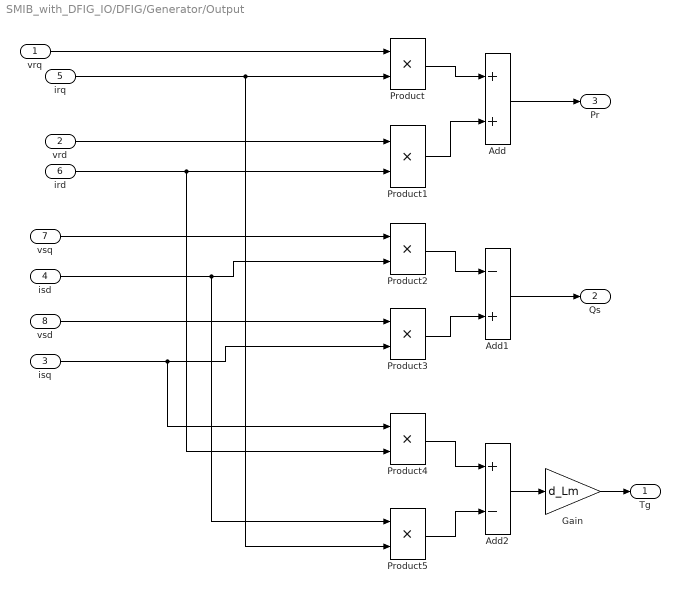
== system SMIB_with_DFIG_IO/DFIG/Generator/Output ==
  vrq : Inport
  vrd : Inport  Port=2
  isq : Inport  Port=3
  isd : Inport  Port=4
  irq : Inport  Port=5
  ird : Inport  Port=6
  vsq : Inport  Port=7
  vsd : Inport  Port=8
  Add : Sum
  Add1 : Sum  Inputs=-+
  Add2 : Sum  Inputs=+-
  Gain : Gain  Gain=d_Lm
  Product{,1..5} (6 alike) : Product
  Tg : Outport
  Qs : Outport  Port=2
  Pr : Outport  Port=3
  wires:
  vrq/1 -> Product/1
  irq/1 -> Product5/2, Product/2
  Product/1 -> Add/1
  Product1/1 -> Add/2
  vrd/1 -> Product1/1
  ird/1 -> Product4/2, Product1/2
  Add/1 -> Pr/1
  Add1/1 -> Qs/1
  Product2/1 -> Add1/1
  Product3/1 -> Add1/2
  Add2/1 -> Gain/1
  Gain/1 -> Tg/1
  Product4/1 -> Add2/1
  Product5/1 -> Add2/2
  vsq/1 -> Product2/1
  isd/1 -> Product5/1, Product2/2
  vsd/1 -> Product3/1
  isq/1 -> Product4/1, Product3/2

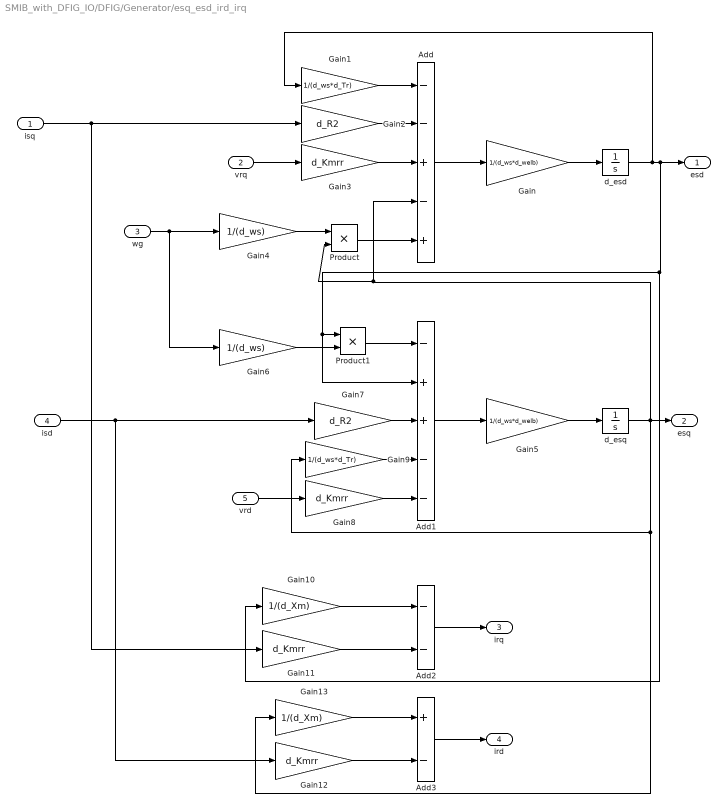
== system SMIB_with_DFIG_IO/DFIG/Generator/esq_esd_ird_irq ==
  isq : Inport
  vrq : Inport  Port=2
  wg : Inport  Port=3
  isd : Inport  Port=4
  vrd : Inport  Port=5
  Add : Sum  Inputs=--+-+
  Add1 : Sum  Inputs=-++--
  Add2 : Sum  Inputs=--
  Add3 : Sum  Inputs=+-
  Gain : Gain  Gain=1/(d_ws*d_welb)
  Gain1 : Gain  Gain=1/(d_ws*d_Tr)
  Gain10 : Gain  Gain=1/(d_Xm)
  Gain{3,8,11..12} (4 alike) : Gain  Gain=d_Kmrr
  Gain13 : Gain  Gain=1/(d_Xm)
  Gain2 : Gain  Gain=d_R2
  Gain4 : Gain  Gain=1/(d_ws)
  Gain5 : Gain  Gain=1/(d_ws*d_welb)
  Gain6 : Gain  Gain=1/(d_ws)
  Gain7 : Gain  Gain=d_R2
  Gain9 : Gain  Gain=1/(d_ws*d_Tr)
  Product : Product
  Product1 : Product
  d_esd : Integrator  InitialCondition=d_esd
  d_esq : Integrator  InitialCondition=d_esq
  esd : Outport
  esq : Outport  Port=2
  irq : Outport  Port=3
  ird : Outport  Port=4
  wires:
  d_esd/1 -> Gain10/1, Add1/2, Product1/1, esd/1, Gain1/1
  Add/1 -> Gain/1
  Gain/1 -> d_esd/1
  Gain1/1 -> Add/1
  Gain2/1 -> Add/2
  Gain3/1 -> Add/3
  vrq/1 -> Gain3/1
  wg/1 -> Gain6/1, Gain4/1
  Gain4/1 -> Product/1
  Product/1 -> Add/5
  Add1/1 -> Gain5/1
  Gain5/1 -> d_esq/1
  d_esq/1 -> Gain13/1, Gain9/1, Product/2, Add/4, esq/1
  Product1/1 -> Add1/1
  Gain6/1 -> Product1/2
  Gain7/1 -> Add1/3
  Gain8/1 -> Add1/5
  vrd/1 -> Gain8/1
  Gain9/1 -> Add1/4
  Add2/1 -> irq/1
  Add3/1 -> ird/1
  Gain10/1 -> Add2/1
  Gain11/1 -> Add2/2
  isq/1 -> Gain11/1, Gain2/1
  Gain12/1 -> Add3/2
  Gain13/1 -> Add3/1
  isd/1 -> Gain12/1, Gain7/1

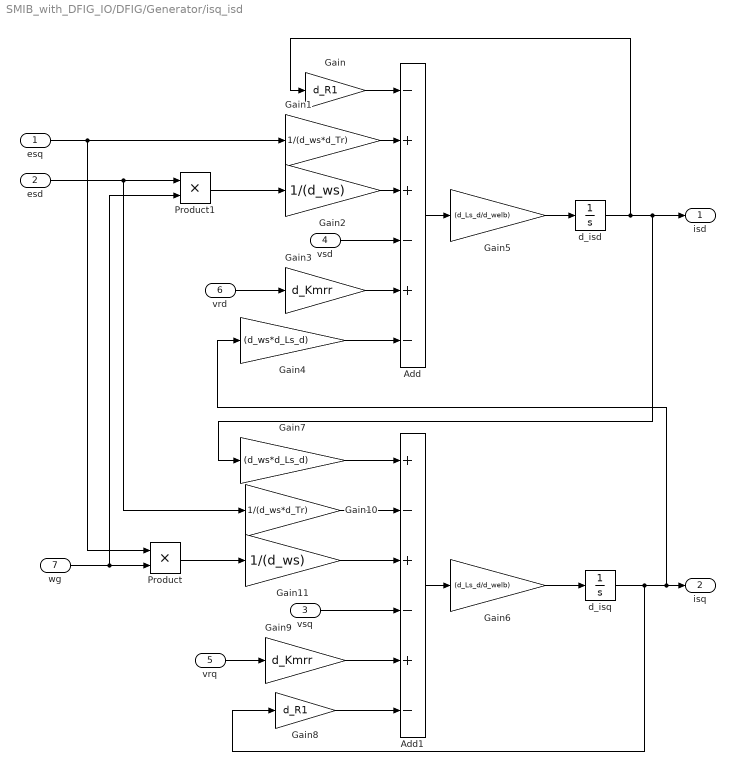
== system SMIB_with_DFIG_IO/DFIG/Generator/isq_isd ==
  esq : Inport
  esd : Inport  Port=2
  vsq : Inport  Port=3
  vsd : Inport  Port=4
  vrq : Inport  Port=5
  vrd : Inport  Port=6
  wg : Inport  Port=7
  Add : Sum  Inputs=-++-+-
  Add1 : Sum  Inputs=+-+-+-
  Gain : Gain  Gain=d_R1
  Gain1 : Gain  Gain=1/(d_ws*d_Tr)
  Gain10 : Gain  Gain=1/(d_ws*d_Tr)
  Gain11 : Gain  Gain=1/(d_ws)
  Gain2 : Gain  Gain=1/(d_ws)
  Gain3 : Gain  Gain=d_Kmrr
  Gain4 : Gain  Gain=(d_ws*d_Ls_d)
  Gain5 : Gain  Gain=(d_Ls_d/d_welb)
  Gain6 : Gain  Gain=(d_Ls_d/d_welb)
  Gain7 : Gain  Gain=(d_ws*d_Ls_d)
  Gain8 : Gain  Gain=d_R1
  Gain9 : Gain  Gain=d_Kmrr
  Product : Product
  Product1 : Product
  d_isd : Integrator  InitialCondition=d_isd
  d_isq : Integrator  InitialCondition=d_isq
  isd : Outport
  isq : Outport  Port=2
  wires:
  d_isd/1 -> Gain7/1, isd/1, Gain/1
  Gain/1 -> Add/1
  esq/1 -> Gain1/1, Product/1
  Gain1/1 -> Add/2
  Gain2/1 -> Add/3
  Gain3/1 -> Add/5
  vrd/1 -> Gain3/1
  Gain4/1 -> Add/6
  Add/1 -> Gain5/1
  Gain5/1 -> d_isd/1
  d_isq/1 -> isq/1, Gain4/1, Gain8/1
  Add1/1 -> Gain6/1
  Gain6/1 -> d_isq/1
  Gain7/1 -> Add1/1
  Gain8/1 -> Add1/6
  Gain9/1 -> Add1/5
  vsq/1 -> Add1/4
  vsd/1 -> Add/4
  vrq/1 -> Gain9/1
  Gain10/1 -> Add1/2
  Gain11/1 -> Add1/3
  Product/1 -> Gain11/1
  Product1/1 -> Gain2/1
  wg/1 -> Product1/2, Product/2
  esd/1 -> Gain10/1, Product1/1

== system SMIB_with_DFIG_IO/DFIG/MSC/MSC_IL1 ==
  In1 : Inport
  Gain : Gain  Gain=d_MSC_IL1_kp
  Gain1 : Gain  Gain=d_MSC_IL1_kp
  Sum : Sum  Inputs=+|+
  d_MSC_IL1_iv : Integrator  InitialCondition=d_MSC_IL1_iv
  vQref : Outport
  wires:
  In1/1 -> Gain1/1, Gain/1
  Gain/1 -> d_MSC_IL1_iv/1
  d_MSC_IL1_iv/1 -> Sum/1
  Sum/1 -> vQref/1
  Gain1/1 -> Sum/2

== system SMIB_with_DFIG_IO/DFIG/MSC/MSC_IL2 ==
  In1 : Inport
  Gain : Gain  Gain=d_MSC_IL2_kp
  Gain1 : Gain  Gain=d_MSC_IL2_kp
  Sum : Sum  Inputs=+|+
  d_MSC_IL2_iv : Integrator  InitialCondition=d_MSC_IL2_iv
  vDref : Outport
  wires:
  In1/1 -> Gain1/1, Gain/1
  Gain/1 -> d_MSC_IL2_iv/1
  d_MSC_IL2_iv/1 -> Sum/1
  Sum/1 -> vDref/1
  Gain1/1 -> Sum/2

== system SMIB_with_DFIG_IO/DFIG/MSC/MSC_OL1 ==
  In1 : Inport
  Gain : Gain  Gain=d_MSC_OL1_kp
  Gain1 : Gain  Gain=d_MSC_OL1_kp
  Sum : Sum  Inputs=+|+
  d_MSC_OL1_iv : Integrator  InitialCondition=d_MSC_OL1_iv
  iQref : Outport
  wires:
  In1/1 -> Gain1/1, Gain/1
  Gain/1 -> d_MSC_OL1_iv/1
  d_MSC_OL1_iv/1 -> Sum/1
  Sum/1 -> iQref/1
  Gain1/1 -> Sum/2

== system SMIB_with_DFIG_IO/DFIG/MSC/MSC_OL2 ==
  In1 : Inport
  Gain : Gain  Gain=d_MSC_OL2_kp
  Gain1 : Gain  Gain=d_MSC_OL2_kp
  Sum : Sum  Inputs=+|+
  d_MSC_OL2_iv : Integrator  InitialCondition=d_MSC_OL2_iv
  iDref : Outport
  wires:
  In1/1 -> Gain1/1, Gain/1
  Gain/1 -> d_MSC_OL2_iv/1
  d_MSC_OL2_iv/1 -> Sum/1
  Sum/1 -> iDref/1
  Gain1/1 -> Sum/2

== system SMIB_with_DFIG_IO/DFIG/MSC/Subsystem ==
  irq : Inport
  ird : Inport  Port=2
  Theta : Inport  Port=3
  Complex to Real-Imag : ComplexToRealImag
  Gain : Gain  Gain=-j
  Math Function : Math  SaturateOnIntegerOverflow=on
  Product : Product
  Real-Imag to Complex : RealImagToComplex
  irq' : Outport
  ird' : Outport  Port=2
  wires:
  irq/1 -> Real-Imag to Complex/1
  ird/1 -> Real-Imag to Complex/2
  Gain/1 -> Math Function/1
  Theta/1 -> Gain/1
  Real-Imag to Complex/1 -> Product/1
  Math Function/1 -> Product/2
  Product/1 -> Complex to Real-Imag/1
  Complex to Real-Imag/1 -> irq'/1
  Complex to Real-Imag/2 -> ird'/1

== system SMIB_with_DFIG_IO/DFIG/MSC/Subsystem1 ==
  vrq' : Inport
  vrd' : Inport  Port=2
  Theta : Inport  Port=3
  Complex to Real-Imag : ComplexToRealImag
  Gain : Gain  Gain=j
  Math Function : Math  SaturateOnIntegerOverflow=on
  Product : Product
  Real-Imag to Complex : RealImagToComplex
  vrq : Outport
  vrd : Outport  Port=2
  wires:
  vrq'/1 -> Real-Imag to Complex/1
  vrd'/1 -> Real-Imag to Complex/2
  Gain/1 -> Math Function/1
  Theta/1 -> Gain/1
  Real-Imag to Complex/1 -> Product/1
  Math Function/1 -> Product/2
  Product/1 -> Complex to Real-Imag/1
  Complex to Real-Imag/1 -> vrq/1
  Complex to Real-Imag/2 -> vrd/1

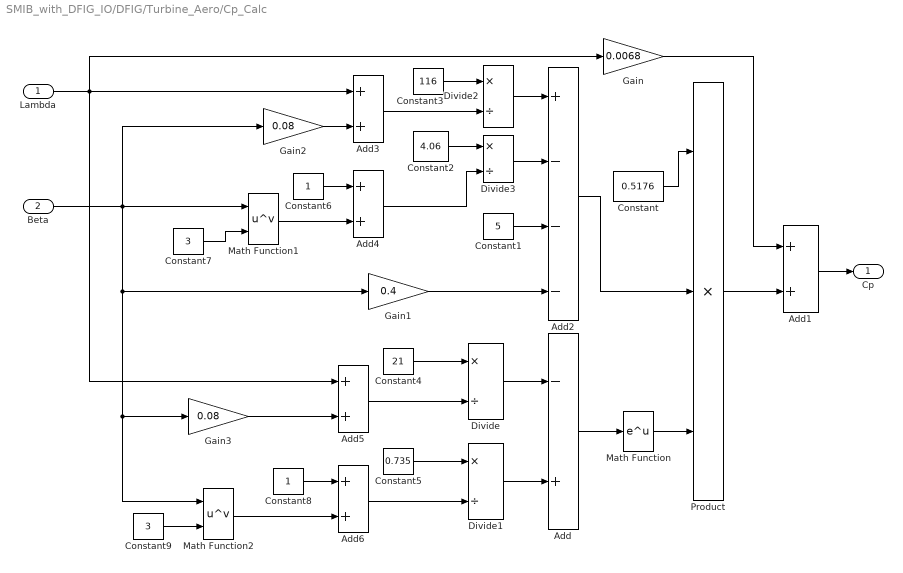
== system SMIB_with_DFIG_IO/DFIG/Turbine_Aero/Cp_Calc ==
  Lambda : Inport
  Beta : Inport  Port=2
  Add : Sum  Inputs=-+
  Add{1,3..6} (5 alike) : Sum
  Add2 : Sum  Inputs=+---
  Constant : Constant  Value=0.5176
  Constant1 : Constant  Value=5
  Constant2 : Constant  Value=4.06
  Constant3 : Constant  Value=116
  Constant4 : Constant  Value=21
  Constant5 : Constant  Value=0.735
  Constant6 : Constant
  Constant7 : Constant  Value=3
  Constant8 : Constant
  Constant9 : Constant  Value=3
  Divide{,1..3} (4 alike) : Product  Inputs=*/
  Gain : Gain  Gain=0.0068
  Gain1 : Gain  Gain=0.4
  Gain2 : Gain  Gain=0.08
  Gain3 : Gain  Gain=0.08
  Math Function : Math  SaturateOnIntegerOverflow=on
  Math Function1 : Math  Operator=pow  SaturateOnIntegerOverflow=on
  Math Function2 : Math  Operator=pow  SaturateOnIntegerOverflow=on
  Product : Product  Inputs=3
  Cp : Outport
  wires:
  Product/1 -> Add1/2
  Add1/1 -> Cp/1
  Gain/1 -> Add1/1
  Constant/1 -> Product/1
  Add/1 -> Math Function/1
  Divide/1 -> Add/1
  Divide1/1 -> Add/2
  Lambda/1 -> Gain/1, Add5/1, Add3/1
  Math Function/1 -> Product/3
  Add2/1 -> Product/2
  Constant1/1 -> Add2/3
  Divide2/1 -> Add2/1
  Divide3/1 -> Add2/2
  Constant2/1 -> Divide3/1
  Constant3/1 -> Divide2/1
  Add3/1 -> Divide2/2
  Add4/1 -> Divide3/2
  Gain1/1 -> Add2/4
  Constant4/1 -> Divide/1
  Add5/1 -> Divide/2
  Add6/1 -> Divide1/2
  Constant5/1 -> Divide1/1
  Gain2/1 -> Add3/2
  Constant6/1 -> Add4/1
  Math Function1/1 -> Add4/2
  Constant7/1 -> Math Function1/2
  Beta/1 -> Gain2/1, Gain1/1, Gain3/1, Math Function2/1, Math Function1/1
  Gain3/1 -> Add5/2
  Constant8/1 -> Add6/1
  Math Function2/1 -> Add6/2
  Constant9/1 -> Math Function2/2

== system SMIB_with_DFIG_IO/SMIB/Machine/DQ to dq ==
  V1 : Inport
  exp(-j*s_delta) : Inport  Port=2
  Complex to Real-Imag : ComplexToRealImag
  Product1 : Product
  "s_vq " : Outport
  s_vd : Outport  Port=2
  wires:
  Complex to Real-Imag/1 -> "s_vq "/1
  Complex to Real-Imag/2 -> s_vd/1
  Product1/1 -> Complex to Real-Imag/1
  V1/1 -> Product1/1
  exp(-j*s_delta)/1 -> Product1/2

== system SMIB_with_DFIG_IO/SMIB/Machine/Machine Equations ==
  s_Efd : Inport
  s_vd : Inport  Port=2
  s_vq : Inport  Port=3
  s_Ed_dash : Subsystem
  s_Eq_dash : Subsystem
  s_I : Subsystem
  s_Psi12q : Subsystem
  s_Psi1d : Subsystem
  "s_Te " : Subsystem
  s_Te : Outport
  s_iq : Outport  Port=2
  s_id : Outport  Port=3
  wires:
  "s_Te "/1(s_Te) -> s_Te/1
  s_Efd/1 -> s_Eq_dash/2(s_Efd)
  s_Eq_dash/1(s_Eq_dash) -> s_Psi1d/2(s_Eq_dash), s_I/2(s_Eq_dash), "s_Te "/2(s_Eq_dash)
  s_I/1(s_id) -> s_Psi1d/1(s_id), "s_Te "/4(s_id), s_Eq_dash/1(s_id), s_id/1
  s_I/2(s_iq) -> "s_Te "/3(s_iq), s_Ed_dash/1(s_iq), s_Psi12q/1(s_iq), s_iq/1
  s_vd/1 -> s_I/3(s_vd)
  s_vq/1 -> s_I/4(s_vq)
  s_Ed_dash/1(s_Ed_dash) -> s_Psi12q/2(s_Ed_dash), s_I/1(s_Ed_dash), "s_Te "/1(s_Ed_dash)
  s_Psi12q/1(s_Psi2q) -> s_I/6(s_Psi2q), "s_Te "/6(s_Psi2q), s_Ed_dash/2(s_Psi2q)
  s_Psi1d/1(s_Psi1d) -> s_I/5(s_Psi1d), s_Eq_dash/3(s_Psi1d), "s_Te "/5(s_Psild)

== system SMIB_with_DFIG_IO/SMIB/Machine/Mathematical block ==
  s_delta : Inport
  Gain1 : Gain  Gain=j
  Gain2 : Gain  Gain=-j
  Math Function1 : Math  SaturateOnIntegerOverflow=on
  Math Function2 : Math  SaturateOnIntegerOverflow=on
  exp(-j*s_delta) : Outport
  exp(j*s_delta) : Outport  Port=2
  wires:
  Gain1/1 -> Math Function1/1
  Gain2/1 -> Math Function2/1
  Math Function1/1 -> exp(j*s_delta)/1
  s_delta/1 -> Gain2/1, Gain1/1
  Math Function2/1 -> exp(-j*s_delta)/1

== system SMIB_with_DFIG_IO/SMIB/Machine/dq to DQ ==
  s_iq : Inport
  s_id : Inport  Port=2
  exp(j*s_delta) : Inport  Port=3
  Product : Product
  Real-Imag to Complex : RealImagToComplex
  s_iDQ : Outport
  wires:
  s_iq/1 -> Real-Imag to Complex/1
  s_id/1 -> Real-Imag to Complex/2
  Real-Imag to Complex/1 -> Product/1
  Product/1 -> s_iDQ/1
  exp(j*s_delta)/1 -> Product/2

== system SMIB_with_DFIG_IO/SMIB/Machine/Machine Equations/s_Ed_dash ==
  s_iq : Inport
  s_Psi2q : Inport  Port=2
  " " : Gain  Gain=s_xq-s_xqd
  "  " : Gain  Gain=(s_xqd-s_xqdd)./((s_xqd-s_xls).^2)
  Add2 : Sum  Inputs=+-
  Add3 : Sum  Inputs=-+
  Add4 : Sum  Inputs=-+-
  Gain : Gain  Gain=1./s_Tqod
  Gain1 : Gain  Gain=s_xqd-s_xls
  s_Edd : Integrator  InitialCondition=s_Edd
  s_Ed_dash : Outport
  wires:
  s_iq/1 -> Gain1/1, Add3/1
  Add3/1 -> " "/1
  " "/1 -> Add2/1
  Gain1/1 -> Add4/2
  s_Psi2q/1 -> Add4/1
  Add2/1 -> Gain/1
  Gain/1 -> s_Edd/1
  s_Edd/1 -> Add2/2, Add4/3, s_Ed_dash/1
  Add4/1 -> "  "/1
  "  "/1 -> Add3/2

== system SMIB_with_DFIG_IO/SMIB/Machine/Machine Equations/s_Eq_dash ==
  s_id : Inport
  s_Efd : Inport  Port=2
  s_Psi1d : Inport  Port=3
  "  " : Gain  Gain=s_xdd-s_xls
  "    " : Gain  Gain=s_xd-s_xdd
  "         " : Gain  Gain=(s_xdd-s_xddd)./((s_xdd-s_xls).^2)
  Add1 : Sum
  Add2 : Sum  Inputs=+-
  Add3 : Sum
  Add4 : Sum  Inputs=+--
  Gain : Gain  Gain=1./s_Tdod
  s_Eqd : Integrator  InitialCondition=s_Eqd
  s_Eq_dash : Outport
  wires:
  s_id/1 -> "  "/1, Add3/1
  Add3/1 -> "    "/1
  "  "/1 -> Add4/2
  s_Psi1d/1 -> Add4/1
  "    "/1 -> Add1/1
  s_Efd/1 -> Add1/2
  Add4/1 -> "         "/1
  "         "/1 -> Add3/2
  Add1/1 -> Add2/1
  Add2/1 -> Gain/1
  Gain/1 -> s_Eqd/1
  s_Eqd/1 -> Add2/2, Add4/3, s_Eq_dash/1

== system SMIB_with_DFIG_IO/SMIB/Machine/Machine Equations/s_I ==
  s_Ed_dash : Inport
  s_Eq_dash : Inport  Port=2
  s_vd : Inport  Port=3
  s_vq : Inport  Port=4
  s_Psi1d : Inport  Port=5
  s_Psi2q : Inport  Port=6
  " " : Sum  Inputs=+-+
  "  " : Gain  Gain=(s_xddd-s_xls)./(s_xdd-s_xls)
  "   " : Gain  Gain=(s_xdd-s_xddd)./(s_xdd-s_xls)
  "    " : Gain  Gain=(s_xqd-s_xqdd)./(s_xqd-s_xls)
  "      " : Sum  Inputs=--+
  "       " : Gain  Gain=(s_xqdd-s_xls)./(s_xqd-s_xls)
  "         " : Sum
  "            " : Sum  Inputs=+-
  Gain1 : Gain  Gain=s_Rs./(s_Rs.^2+s_xddd.^2)
  Gain2 : Gain  Gain=s_xddd./(s_Rs.^2+s_xddd.^2)
  Gain7 : Gain  Gain=s_Rs./(s_Rs.^2+s_xddd.^2)
  Gain8 : Gain  Gain=s_xddd./(s_Rs.^2+s_xddd.^2)
  s_id : Outport
  s_iq : Outport  Port=2
  wires:
  s_Eq_dash/1 -> "  "/1
  s_Psi1d/1 -> "   "/1
  s_vq/1 -> " "/2
  "  "/1 -> " "/1
  "   "/1 -> " "/3
  s_Psi2q/1 -> "    "/1
  "       "/1 -> "      "/3
  s_vd/1 -> "      "/2
  s_Ed_dash/1 -> "       "/1
  " "/1 -> Gain8/1, Gain1/1
  "      "/1 -> Gain7/1, Gain2/1
  Gain1/1 -> "         "/1
  Gain2/1 -> "         "/2
  Gain7/1 -> "            "/1
  Gain8/1 -> "            "/2
  "         "/1 -> s_iq/1
  "            "/1 -> s_id/1
  "    "/1 -> "      "/1

== system SMIB_with_DFIG_IO/SMIB/Machine/Machine Equations/s_Psi12q ==
  s_iq : Inport
  s_Ed_dash : Inport  Port=2
  " " : Gain  Gain=s_xqd-s_xls
  " Gain" : Gain  Gain=1./s_Tqodd
  Add2 : Sum  Inputs=+--
  s_Psi2_q : Integrator  InitialCondition=s_Psi2q
  s_Psi2q : Outport
  wires:
  s_iq/1 -> " "/1
  " "/1 -> Add2/1
  s_Ed_dash/1 -> Add2/2
  Add2/1 -> " Gain"/1
  " Gain"/1 -> s_Psi2_q/1
  s_Psi2_q/1 -> Add2/3, s_Psi2q/1

== system SMIB_with_DFIG_IO/SMIB/Machine/Machine Equations/s_Psi1d ==
  s_id : Inport
  s_Eq_dash : Inport  Port=2
  " " : Gain  Gain=s_xdd-s_xls
  Add2 : Sum  Inputs=++-
  Gain : Gain  Gain=1./s_Tdodd
  s_Psi1_d : Integrator  InitialCondition=s_Psild
  s_Psi1d : Outport
  wires:
  s_id/1 -> " "/1
  " "/1 -> Add2/1
  s_Eq_dash/1 -> Add2/2
  Add2/1 -> Gain/1
  Gain/1 -> s_Psi1_d/1
  s_Psi1_d/1 -> Add2/3, s_Psi1d/1

== system SMIB_with_DFIG_IO/SMIB/Machine/Machine Equations/s_Te  ==
  s_Ed_dash : Inport
  s_Eq_dash : Inport  Port=2
  s_iq : Inport  Port=3
  s_id : Inport  Port=4
  s_Psild : Inport  Port=5
  s_Psi2q : Inport  Port=6
  Add3 : Sum  Inputs=++++-
  Gain : Gain  Gain=(s_xqdd-s_xls)./(s_xqd-s_xls)
  Gain1 : Gain  Gain=(s_xddd-s_xls)./(s_xdd-s_xls)
  Gain2 : Gain  Gain=s_xqdd-s_xddd
  Gain3 : Gain  Gain=(s_xdd-s_xddd)./(s_xdd-s_xls)
  Gain4 : Gain  Gain=(s_xqd-s_xqdd)./(s_xqd-s_xls)
  Product{,1..4} (5 alike) : Product
  s_Te : Outport
  wires:
  s_Ed_dash/1 -> Product/1
  Product/1 -> Gain/1
  Product1/1 -> Gain1/1
  Product2/1 -> Gain2/1
  Product3/1 -> Gain3/1
  Product4/1 -> Gain4/1
  Gain/1 -> Add3/1
  Gain1/1 -> Add3/2
  Gain2/1 -> Add3/3
  Gain3/1 -> Add3/4
  Gain4/1 -> Add3/5
  s_Psi2q/1 -> Product4/1
  s_Psild/1 -> Product3/1
  s_iq/1 -> Product3/2, Product1/2, Product2/2
  s_Eq_dash/1 -> Product1/1
  s_id/1 -> Product/2, Product4/2, Product2/1
  Add3/1 -> s_Te/1
